simulink model "SIFT_final"  (R2015a)
settings: Solver=ode45  StartTime=0.0  StopTime=10.0  RelTol=1e-3
InitFcn:
  | %% DSPBuilder Start
  | alt_dspbuilder_update_model(bdroot)
  | %% DSPBuilder End
libraries: allblocks_alteradspbuilder2 x1826
(part 15 of 24)

== system SIFT_final/SIFT/SIFT_detector/Octave0/calculate_key_point/find_KeyPoint/find_Keymax ==
  dataIn_10 : Inport
  dataIn_11 : Inport  Port=2
  dataIn_12 : Inport  Port=3
  dataIn_13 : Inport  Port=4
  dataIn_14 : Inport  Port=5
  dataIn_15 : Inport  Port=6
  dataIn_16 : Inport  Port=7
  dataIn_17 : Inport  Port=8
  dataIn_18 : Inport  Port=9
  dataIn_20 : Inport  Port=10
  dataIn_21 : Inport  Port=11
  dataIn_22 : Inport  Port=12
  dataIn_23 : Inport  Port=13
  dataIn_24 : Inport  Port=14
  dataIn_25 : Inport  Port=15
  dataIn_26 : Inport  Port=16
  dataIn_27 : Inport  Port=17
  dataIn_28 : Inport  Port=18
  dataIn_30 : Inport  Port=19
  dataIn_31 : Inport  Port=20
  dataIn_32 : Inport  Port=21
  dataIn_33 : Inport  Port=22
  dataIn_34 : Inport  Port=23
  dataIn_35 : Inport  Port=24
  dataIn_36 : Inport  Port=25
  dataIn_37 : Inport  Port=26
  dataIn_38 : Inport  Port=27
  Comparator : allblocks_alteradspbuilder2/Comparator  direction=a > b  pipeline_display=0  allowFloatingPointOverride=on  logOutputs=off  logFile=G:\Project\SIFT 2octave\add frb\PCIE_Display\custom_ip\tb_SIFT\SIFT_SIFT_Subsystem_calculate%5Fkey%5Fpoint_find%5FKeyPoint_find%5FKeymax_Comparator.fixedpointlog
  Comparator1 : allblocks_alteradspbuilder2/Comparator  direction=a > b  pipeline_display=0  allowFloatingPointOverride=on  logOutputs=off  logFile=G:\Project\SIFT 2octave\add frb\PCIE_Display\custom_ip\tb_SIFT\SIFT_SIFT_Subsystem_calculate%5Fkey%5Fpoint_find%5FKeyPoint_find%5FKeymax_Comparator1.fixedpointlog
  Comparator10 : allblocks_alteradspbuilder2/Comparator  direction=a > b  pipeline_display=0  allowFloatingPointOverride=on  logOutputs=off  logFile=G:\Project\SIFT 2octave\add frb\PCIE_Display\custom_ip\tb_SIFT\SIFT_SIFT_Subsystem_calculate%5Fkey%5Fpoint_find%5FKeyPoint_find%5FKeymax_Comparator10.fixedpointlog
  Comparator11 : allblocks_alteradspbuilder2/Comparator  direction=a > b  pipeline_display=0  allowFloatingPointOverride=on  logOutputs=off  logFile=G:\Project\SIFT 2octave\add frb\PCIE_Display\custom_ip\tb_SIFT\SIFT_SIFT_Subsystem_calculate%5Fkey%5Fpoint_find%5FKeyPoint_find%5FKeymax_Comparator11.fixedpointlog
  Comparator12 : allblocks_alteradspbuilder2/Comparator  direction=a > b  pipeline_display=0  allowFloatingPointOverride=on  logOutputs=off  logFile=G:\Project\SIFT 2octave\add frb\PCIE_Display\custom_ip\tb_SIFT\SIFT_SIFT_Subsystem_calculate%5Fkey%5Fpoint_find%5FKeyPoint_find%5FKeymax_Comparator12.fixedpointlog
  Comparator13 : allblocks_alteradspbuilder2/Comparator  direction=a > b  pipeline_display=0  allowFloatingPointOverride=on  logOutputs=off  logFile=G:\Project\SIFT 2octave\add frb\PCIE_Display\custom_ip\tb_SIFT\SIFT_SIFT_Subsystem_calculate%5Fkey%5Fpoint_find%5FKeyPoint_find%5FKeymax_Comparator13.fixedpointlog
  Comparator14 : allblocks_alteradspbuilder2/Comparator  direction=a > b  pipeline_display=0  allowFloatingPointOverride=on  logOutputs=off  logFile=G:\Project\SIFT 2octave\add frb\PCIE_Display\custom_ip\tb_SIFT\SIFT_SIFT_Subsystem_calculate%5Fkey%5Fpoint_find%5FKeyPoint_find%5FKeymax_Comparator14.fixedpointlog
  Comparator15 : allblocks_alteradspbuilder2/Comparator  direction=a > b  pipeline_display=0  allowFloatingPointOverride=on  logOutputs=off  logFile=G:\Project\SIFT 2octave\add frb\PCIE_Display\custom_ip\tb_SIFT\SIFT_SIFT_Subsystem_calculate%5Fkey%5Fpoint_find%5FKeyPoint_find%5FKeymax_Comparator15.fixedpointlog
  Comparator16 : allblocks_alteradspbuilder2/Comparator  direction=a > b  pipeline_display=0  allowFloatingPointOverride=on  logOutputs=off  logFile=G:\Project\SIFT 2octave\add frb\PCIE_Display\custom_ip\tb_SIFT\SIFT_SIFT_Subsystem_calculate%5Fkey%5Fpoint_find%5FKeyPoint_find%5FKeymax_Comparator16.fixedpointlog
  Comparator17 : allblocks_alteradspbuilder2/Comparator  direction=a > b  pipeline_display=0  allowFloatingPointOverride=on  logOutputs=off  logFile=G:\Project\SIFT 2octave\add frb\PCIE_Display\custom_ip\tb_SIFT\SIFT_SIFT_Subsystem_calculate%5Fkey%5Fpoint_find%5FKeyPoint_find%5FKeymax_Comparator17.fixedpointlog
  Comparator19 : allblocks_alteradspbuilder2/Comparator  direction=a > b  pipeline_display=0  allowFloatingPointOverride=on  logOutputs=off  logFile=G:\Project\SIFT 2octave\add frb\PCIE_Display\custom_ip\tb_SIFT\SIFT_SIFT_Subsystem_calculate%5Fkey%5Fpoint_find%5FKeyPoint_find%5FKeymax_Comparator19.fixedpointlog
  Comparator2 : allblocks_alteradspbuilder2/Comparator  direction=a > b  pipeline_display=0  allowFloatingPointOverride=on  logOutputs=off  logFile=G:\Project\SIFT 2octave\add frb\PCIE_Display\custom_ip\tb_SIFT\SIFT_SIFT_Subsystem_calculate%5Fkey%5Fpoint_find%5FKeyPoint_find%5FKeymax_Comparator2.fixedpointlog
  Comparator20 : allblocks_alteradspbuilder2/Comparator  direction=a > b  pipeline_display=0  allowFloatingPointOverride=on  logOutputs=off  logFile=G:\Project\SIFT 2octave\add frb\PCIE_Display\custom_ip\tb_SIFT\SIFT_SIFT_Subsystem_calculate%5Fkey%5Fpoint_find%5FKeyPoint_find%5FKeymax_Comparator20.fixedpointlog
  Comparator27 : allblocks_alteradspbuilder2/Comparator  direction=a > b  pipeline_display=0  allowFloatingPointOverride=on  logOutputs=off  logFile=G:\Project\SIFT 2octave\add frb\PCIE_Display\custom_ip\tb_SIFT\SIFT_SIFT_Subsystem_calculate%5Fkey%5Fpoint_find%5FKeyPoint_find%5FKeymax_Comparator27.fixedpointlog
  Comparator28 : allblocks_alteradspbuilder2/Comparator  direction=a > b  pipeline_display=0  allowFloatingPointOverride=on  logOutputs=off  logFile=G:\Project\SIFT 2octave\add frb\PCIE_Display\custom_ip\tb_SIFT\SIFT_SIFT_Subsystem_calculate%5Fkey%5Fpoint_find%5FKeyPoint_find%5FKeymax_Comparator28.fixedpointlog
  Comparator29 : allblocks_alteradspbuilder2/Comparator  direction=a > b  pipeline_display=0  allowFloatingPointOverride=on  logOutputs=off  logFile=G:\Project\SIFT 2octave\add frb\PCIE_Display\custom_ip\tb_SIFT\SIFT_SIFT_Subsystem_calculate%5Fkey%5Fpoint_find%5FKeyPoint_find%5FKeymax_Comparator29.fixedpointlog
  Comparator3 : allblocks_alteradspbuilder2/Comparator  direction=a > b  pipeline_display=0  allowFloatingPointOverride=on  logOutputs=off  logFile=G:\Project\SIFT 2octave\add frb\PCIE_Display\custom_ip\tb_SIFT\SIFT_SIFT_Subsystem_calculate%5Fkey%5Fpoint_find%5FKeyPoint_find%5FKeymax_Comparator3.fixedpointlog
  Comparator30 : allblocks_alteradspbuilder2/Comparator  direction=a > b  pipeline_display=0  allowFloatingPointOverride=on  logOutputs=off  logFile=G:\Project\SIFT 2octave\add frb\PCIE_Display\custom_ip\tb_SIFT\SIFT_SIFT_Subsystem_calculate%5Fkey%5Fpoint_find%5FKeyPoint_find%5FKeymax_Comparator30.fixedpointlog
  Comparator31 : allblocks_alteradspbuilder2/Comparator  direction=a > b  pipeline_display=0  allowFloatingPointOverride=on  logOutputs=off  logFile=G:\Project\SIFT 2octave\add frb\PCIE_Display\custom_ip\tb_SIFT\SIFT_SIFT_Subsystem_calculate%5Fkey%5Fpoint_find%5FKeyPoint_find%5FKeymax_Comparator31.fixedpointlog
  Comparator32 : allblocks_alteradspbuilder2/Comparator  direction=a > b  pipeline_display=0  allowFloatingPointOverride=on  logOutputs=off  logFile=G:\Project\SIFT 2octave\add frb\PCIE_Display\custom_ip\tb_SIFT\SIFT_SIFT_Subsystem_calculate%5Fkey%5Fpoint_find%5FKeyPoint_find%5FKeymax_Comparator32.fixedpointlog
  Comparator33 : allblocks_alteradspbuilder2/Comparator  direction=a > b  pipeline_display=0  allowFloatingPointOverride=on  logOutputs=off  logFile=G:\Project\SIFT 2octave\add frb\PCIE_Display\custom_ip\tb_SIFT\SIFT_SIFT_Subsystem_calculate%5Fkey%5Fpoint_find%5FKeyPoint_find%5FKeymax_Comparator33.fixedpointlog
  Comparator34 : allblocks_alteradspbuilder2/Comparator  direction=a > b  pipeline_display=0  allowFloatingPointOverride=on  logOutputs=off  logFile=G:\Project\SIFT 2octave\add frb\PCIE_Display\custom_ip\tb_SIFT\SIFT_SIFT_Subsystem_calculate%5Fkey%5Fpoint_find%5FKeyPoint_find%5FKeymax_Comparator34.fixedpointlog
  Comparator35 : allblocks_alteradspbuilder2/Comparator  direction=a > b  pipeline_display=0  allowFloatingPointOverride=on  logOutputs=off  logFile=G:\Project\SIFT 2octave\add frb\PCIE_Display\custom_ip\tb_SIFT\SIFT_SIFT_Subsystem_calculate%5Fkey%5Fpoint_find%5FKeyPoint_find%5FKeymax_Comparator35.fixedpointlog
  Comparator4 : allblocks_alteradspbuilder2/Comparator  direction=a > b  pipeline_display=0  allowFloatingPointOverride=on  logOutputs=off  logFile=G:\Project\SIFT 2octave\add frb\PCIE_Display\custom_ip\tb_SIFT\SIFT_SIFT_Subsystem_calculate%5Fkey%5Fpoint_find%5FKeyPoint_find%5FKeymax_Comparator4.fixedpointlog
  Comparator5 : allblocks_alteradspbuilder2/Comparator  direction=a > b  pipeline_display=0  allowFloatingPointOverride=on  logOutputs=off  logFile=G:\Project\SIFT 2octave\add frb\PCIE_Display\custom_ip\tb_SIFT\SIFT_SIFT_Subsystem_calculate%5Fkey%5Fpoint_find%5FKeyPoint_find%5FKeymax_Comparator5.fixedpointlog
  Comparator6 : allblocks_alteradspbuilder2/Comparator  direction=a < b  pipeline_display=0  allowFloatingPointOverride=on  logOutputs=off  logFile=G:\Project\SIFT 2octave\add frb\PCIE_Display\custom_ip\tb_SIFT\SIFT_SIFT_Subsystem_calculate%5Fkey%5Fpoint_find%5FKeyPoint_find%5FKeymax_Comparator6.fixedpointlog
  Comparator7 : allblocks_alteradspbuilder2/Comparator  direction=a < b  pipeline_display=0  allowFloatingPointOverride=on  logOutputs=off  logFile=G:\Project\SIFT 2octave\add frb\PCIE_Display\custom_ip\tb_SIFT\SIFT_SIFT_Subsystem_calculate%5Fkey%5Fpoint_find%5FKeyPoint_find%5FKeymax_Comparator7.fixedpointlog
  Comparator9 : allblocks_alteradspbuilder2/Comparator  direction=a > b  pipeline_display=0  allowFloatingPointOverride=on  logOutputs=off  logFile=G:\Project\SIFT 2octave\add frb\PCIE_Display\custom_ip\tb_SIFT\SIFT_SIFT_Subsystem_calculate%5Fkey%5Fpoint_find%5FKeyPoint_find%5FKeymax_Comparator9.fixedpointlog
  Constant : allblocks_alteradspbuilder2/Constant  mask_cst=0.8*0.015  BusType=Signed Fractional  bwl=9  bwr=16  roundMode=Truncate  satMode=Wrap  SpecifyClock=off  allowFloatingPointOverride=on  logOutputs=off  logFile=G:\Project\SIFT 2octave\add frb\PCIE_Display\custom_ip\tb_SIFT\SIFT_SIFT_Subsystem_calculate%5Fkey%5Fpoint_find%5FKeyPoint_find%5FKeymax_Constant.fixedpointlog
  Constant1 : allblocks_alteradspbuilder2/Constant  mask_cst=-0.8*0.015  BusType=Signed Fractional  bwl=9  bwr=16  roundMode=Truncate  satMode=Wrap  SpecifyClock=off  allowFloatingPointOverride=on  logOutputs=off  logFile=G:\Project\SIFT 2octave\add frb\PCIE_Display\custom_ip\tb_SIFT\SIFT_SIFT_Subsystem_calculate%5Fkey%5Fpoint_find%5FKeyPoint_find%5FKeymax_Constant1.fixedpointlog
  Logical Bit Operator : allblocks_alteradspbuilder2/Logical Bit Operator  LogicalOperator=OR  user_inputs=2  pipeline_display=0
  Logical Bit Operator2 : allblocks_alteradspbuilder2/Logical Bit Operator  LogicalOperator=AND  user_inputs=27  pipeline_display=0
  is_KeyPoint : Outport
  wires:
  dataIn_18/1 -> [dataIn_18]
  dataIn_10/1 -> [dataIn_10]
  [result_10] -> Logical Bit Operator2/1
  [dataIn_24] -> Comparator/1
  Comparator1/1 -> [result_11]
  [dataIn_10] -> Comparator/2
  [dataIn_24] -> Comparator1/1
  [dataIn_11] -> Comparator1/2
  [result_20] -> Logical Bit Operator2/10
  [result_11] -> Logical Bit Operator2/2
  [result_22] -> Logical Bit Operator2/12
  [result_23] -> Logical Bit Operator2/13
  Comparator7/1 -> Logical Bit Operator/2
  [dataIn_24] -> Comparator2/1
  [dataIn_24] -> Comparator6/2
  Comparator2/1 -> [result_12]
  [dataIn_12] -> Comparator2/2
  [result_21] -> Logical Bit Operator2/11
  [dataIn_24] -> Comparator9/1
  Comparator9/1 -> [result_16]
  [dataIn_24] -> Comparator10/1
  [dataIn_16] -> Comparator9/2
  Comparator10/1 -> [result_17]
  [dataIn_17] -> Comparator10/2
  [dataIn_24] -> Comparator11/1
  Comparator11/1 -> [result_18]
  [dataIn_18] -> Comparator11/2
  dataIn_14/1 -> [dataIn_14]
  dataIn_15/1 -> [dataIn_15]
  dataIn_17/1 -> [dataIn_17]
  dataIn_16/1 -> [dataIn_16]
  dataIn_24/1 -> [dataIn_24]
  dataIn_27/1 -> [dataIn_27]
  dataIn_28/1 -> [dataIn_28]
  dataIn_25/1 -> [dataIn_25]
  dataIn_22/1 -> [dataIn_22]
  dataIn_20/1 -> [dataIn_20]
  dataIn_21/1 -> [dataIn_21]
  dataIn_23/1 -> [dataIn_23]
  dataIn_26/1 -> [dataIn_26]
  dataIn_30/1 -> [dataIn_30]
  dataIn_31/1 -> [dataIn_31]
  dataIn_32/1 -> [dataIn_32]
  dataIn_33/1 -> [dataIn_33]
  dataIn_37/1 -> [dataIn_37]
  dataIn_35/1 -> [dataIn_35]
  dataIn_34/1 -> [dataIn_34]
  dataIn_36/1 -> [dataIn_36]
  dataIn_38/1 -> [dataIn_38]
  dataIn_11/1 -> [dataIn_11]
  [dataIn_24] -> Comparator7/1
  [dataIn_13] -> Comparator3/2
  Comparator3/1 -> [result_13]
  [dataIn_24] -> Comparator4/1
  [dataIn_24] -> Comparator3/1
  [dataIn_24] -> Comparator5/1
  Comparator5/1 -> [result_15]
  [dataIn_14] -> Comparator4/2
  [dataIn_15] -> Comparator5/2
  Comparator4/1 -> [result_14]
  [dataIn_24] -> Comparator27/1
  [dataIn_24] -> Comparator28/1
  [dataIn_24] -> Comparator31/1
  [dataIn_32] -> Comparator31/2
  [dataIn_24] -> Comparator32/1
  [dataIn_33] -> Comparator32/2
  [dataIn_24] -> Comparator33/1
  Comparator32/1 -> [result_33]
  Comparator27/1 -> [result_30]
  Comparator28/1 -> [result_31]
  Comparator31/1 -> [result_32]
  [dataIn_30] -> Comparator27/2
  [dataIn_31] -> Comparator28/2
  [dataIn_35] -> Comparator34/2
  Comparator35/1 -> [result_36]
  Comparator34/1 -> [result_35]
  [dataIn_34] -> Comparator33/2
  [dataIn_24] -> Comparator35/1
  Comparator29/1 -> [result_37]
  [dataIn_24] -> Comparator30/1
  [dataIn_36] -> Comparator35/2
  Comparator30/1 -> [result_38]
  [dataIn_24] -> Comparator34/1
  [dataIn_24] -> Comparator29/1
  [dataIn_37] -> Comparator29/2
  [dataIn_38] -> Comparator30/2
  Comparator33/1 -> [result_34]
  [result_13] -> Logical Bit Operator2/4
  [result_17] -> Logical Bit Operator2/8
  [result_14] -> Logical Bit Operator2/5
  [result_15] -> Logical Bit Operator2/6
  [result_16] -> Logical Bit Operator2/7
  [result_18] -> Logical Bit Operator2/9
  [result_12] -> Logical Bit Operator2/3
  Constant/1 -> Comparator6/1
  Logical Bit Operator/1 -> [result_24]
  Logical Bit Operator2/1 -> [isKeyPoint]
  Constant1/1 -> Comparator7/2
  Comparator6/1 -> Logical Bit Operator/1
  [dataIn_24] -> Comparator12/1
  [dataIn_25] -> Comparator19/2
  Comparator13/1 -> [result_21]
  Comparator19/1 -> [result_25]
  [dataIn_24] -> Comparator19/1
  [dataIn_20] -> Comparator12/2
  [dataIn_24] -> Comparator16/1
  [dataIn_24] -> Comparator14/1
  [dataIn_24] -> Comparator13/1
  Comparator16/1 -> [result_22]
  [dataIn_22] -> Comparator16/2
  Comparator14/1 -> [result_27]
  [dataIn_24] -> Comparator17/1
  [dataIn_23] -> Comparator17/2
  [dataIn_24] -> Comparator15/1
  [dataIn_27] -> Comparator14/2
  Comparator17/1 -> [result_23]
  [dataIn_28] -> Comparator15/2
  [dataIn_26] -> Comparator20/2
  Comparator12/1 -> [result_20]
  [dataIn_24] -> Comparator20/1
  Comparator15/1 -> [result_28]
  Comparator20/1 -> [result_26]
  [dataIn_21] -> Comparator13/2
  [isKeyPoint] -> is_KeyPoint/1
  dataIn_12/1 -> [dataIn_12]
  dataIn_13/1 -> [dataIn_13]
  Comparator/1 -> [result_10]
  [result_28] -> Logical Bit Operator2/18
  [result_30] -> Logical Bit Operator2/19
  [result_31] -> Logical Bit Operator2/20
  [result_33] -> Logical Bit Operator2/22
  [result_34] -> Logical Bit Operator2/23
  [result_36] -> Logical Bit Operator2/25
  [result_35] -> Logical Bit Operator2/24
  [result_32] -> Logical Bit Operator2/21
  [result_37] -> Logical Bit Operator2/26
  [result_38] -> Logical Bit Operator2/27
  [result_26] -> Logical Bit Operator2/16
  [result_25] -> Logical Bit Operator2/15
  [result_27] -> Logical Bit Operator2/17
  [result_24] -> Logical Bit Operator2/14

== system SIFT_final/SIFT/SIFT_detector/Octave0/calculate_key_point/find_KeyPoint/find_min ==
  dataIn_10 : Inport
  dataIn_11 : Inport  Port=2
  dataIn_12 : Inport  Port=3
  dataIn_13 : Inport  Port=4
  dataIn_14 : Inport  Port=5
  dataIn_15 : Inport  Port=6
  dataIn_16 : Inport  Port=7
  dataIn_17 : Inport  Port=8
  dataIn_18 : Inport  Port=9
  dataIn_20 : Inport  Port=10
  dataIn_21 : Inport  Port=11
  dataIn_22 : Inport  Port=12
  dataIn_23 : Inport  Port=13
  dataIn_24 : Inport  Port=14
  dataIn_25 : Inport  Port=15
  dataIn_26 : Inport  Port=16
  dataIn_27 : Inport  Port=17
  dataIn_28 : Inport  Port=18
  dataIn_30 : Inport  Port=19
  dataIn_31 : Inport  Port=20
  dataIn_32 : Inport  Port=21
  dataIn_33 : Inport  Port=22
  dataIn_34 : Inport  Port=23
  dataIn_35 : Inport  Port=24
  dataIn_36 : Inport  Port=25
  dataIn_37 : Inport  Port=26
  dataIn_38 : Inport  Port=27
  Comparator : allblocks_alteradspbuilder2/Comparator  direction=a < b  pipeline_display=0  allowFloatingPointOverride=on  logOutputs=off  logFile=G:\Project\SIFT 2octave\add frb\PCIE_Display\custom_ip\tb_SIFT\SIFT_SIFT_Subsystem_calculate%5Fkey%5Fpoint_find%5FKeyPoint_find%5Fmin_Comparator.fixedpointlog
  Comparator1 : allblocks_alteradspbuilder2/Comparator  direction=a < b  pipeline_display=0  allowFloatingPointOverride=on  logOutputs=off  logFile=G:\Project\SIFT 2octave\add frb\PCIE_Display\custom_ip\tb_SIFT\SIFT_SIFT_Subsystem_calculate%5Fkey%5Fpoint_find%5FKeyPoint_find%5Fmin_Comparator1.fixedpointlog
  Comparator10 : allblocks_alteradspbuilder2/Comparator  direction=a < b  pipeline_display=0  allowFloatingPointOverride=on  logOutputs=off  logFile=G:\Project\SIFT 2octave\add frb\PCIE_Display\custom_ip\tb_SIFT\SIFT_SIFT_Subsystem_calculate%5Fkey%5Fpoint_find%5FKeyPoint_find%5Fmin_Comparator10.fixedpointlog
  Comparator11 : allblocks_alteradspbuilder2/Comparator  direction=a < b  pipeline_display=0  allowFloatingPointOverride=on  logOutputs=off  logFile=G:\Project\SIFT 2octave\add frb\PCIE_Display\custom_ip\tb_SIFT\SIFT_SIFT_Subsystem_calculate%5Fkey%5Fpoint_find%5FKeyPoint_find%5Fmin_Comparator11.fixedpointlog
  Comparator12 : allblocks_alteradspbuilder2/Comparator  direction=a < b  pipeline_display=0  allowFloatingPointOverride=on  logOutputs=off  logFile=G:\Project\SIFT 2octave\add frb\PCIE_Display\custom_ip\tb_SIFT\SIFT_SIFT_Subsystem_calculate%5Fkey%5Fpoint_find%5FKeyPoint_find%5Fmin_Comparator12.fixedpointlog
  Comparator13 : allblocks_alteradspbuilder2/Comparator  direction=a < b  pipeline_display=0  allowFloatingPointOverride=on  logOutputs=off  logFile=G:\Project\SIFT 2octave\add frb\PCIE_Display\custom_ip\tb_SIFT\SIFT_SIFT_Subsystem_calculate%5Fkey%5Fpoint_find%5FKeyPoint_find%5Fmin_Comparator13.fixedpointlog
  Comparator14 : allblocks_alteradspbuilder2/Comparator  direction=a < b  pipeline_display=0  allowFloatingPointOverride=on  logOutputs=off  logFile=G:\Project\SIFT 2octave\add frb\PCIE_Display\custom_ip\tb_SIFT\SIFT_SIFT_Subsystem_calculate%5Fkey%5Fpoint_find%5FKeyPoint_find%5Fmin_Comparator14.fixedpointlog
  Comparator15 : allblocks_alteradspbuilder2/Comparator  direction=a < b  pipeline_display=0  allowFloatingPointOverride=on  logOutputs=off  logFile=G:\Project\SIFT 2octave\add frb\PCIE_Display\custom_ip\tb_SIFT\SIFT_SIFT_Subsystem_calculate%5Fkey%5Fpoint_find%5FKeyPoint_find%5Fmin_Comparator15.fixedpointlog
  Comparator16 : allblocks_alteradspbuilder2/Comparator  direction=a < b  pipeline_display=0  allowFloatingPointOverride=on  logOutputs=off  logFile=G:\Project\SIFT 2octave\add frb\PCIE_Display\custom_ip\tb_SIFT\SIFT_SIFT_Subsystem_calculate%5Fkey%5Fpoint_find%5FKeyPoint_find%5Fmin_Comparator16.fixedpointlog
  Comparator17 : allblocks_alteradspbuilder2/Comparator  direction=a < b  pipeline_display=0  allowFloatingPointOverride=on  logOutputs=off  logFile=G:\Project\SIFT 2octave\add frb\PCIE_Display\custom_ip\tb_SIFT\SIFT_SIFT_Subsystem_calculate%5Fkey%5Fpoint_find%5FKeyPoint_find%5Fmin_Comparator17.fixedpointlog
  Comparator19 : allblocks_alteradspbuilder2/Comparator  direction=a < b  pipeline_display=0  allowFloatingPointOverride=on  logOutputs=off  logFile=G:\Project\SIFT 2octave\add frb\PCIE_Display\custom_ip\tb_SIFT\SIFT_SIFT_Subsystem_calculate%5Fkey%5Fpoint_find%5FKeyPoint_find%5Fmin_Comparator19.fixedpointlog
  Comparator2 : allblocks_alteradspbuilder2/Comparator  direction=a < b  pipeline_display=0  allowFloatingPointOverride=on  logOutputs=off  logFile=G:\Project\SIFT 2octave\add frb\PCIE_Display\custom_ip\tb_SIFT\SIFT_SIFT_Subsystem_calculate%5Fkey%5Fpoint_find%5FKeyPoint_find%5Fmin_Comparator2.fixedpointlog
  Comparator20 : allblocks_alteradspbuilder2/Comparator  direction=a < b  pipeline_display=0  allowFloatingPointOverride=on  logOutputs=off  logFile=G:\Project\SIFT 2octave\add frb\PCIE_Display\custom_ip\tb_SIFT\SIFT_SIFT_Subsystem_calculate%5Fkey%5Fpoint_find%5FKeyPoint_find%5Fmin_Comparator20.fixedpointlog
  Comparator27 : allblocks_alteradspbuilder2/Comparator  direction=a < b  pipeline_display=0  allowFloatingPointOverride=on  logOutputs=off  logFile=G:\Project\SIFT 2octave\add frb\PCIE_Display\custom_ip\tb_SIFT\SIFT_SIFT_Subsystem_calculate%5Fkey%5Fpoint_find%5FKeyPoint_find%5Fmin_Comparator27.fixedpointlog
  Comparator28 : allblocks_alteradspbuilder2/Comparator  direction=a < b  pipeline_display=0  allowFloatingPointOverride=on  logOutputs=off  logFile=G:\Project\SIFT 2octave\add frb\PCIE_Display\custom_ip\tb_SIFT\SIFT_SIFT_Subsystem_calculate%5Fkey%5Fpoint_find%5FKeyPoint_find%5Fmin_Comparator28.fixedpointlog
  Comparator29 : allblocks_alteradspbuilder2/Comparator  direction=a < b  pipeline_display=0  allowFloatingPointOverride=on  logOutputs=off  logFile=G:\Project\SIFT 2octave\add frb\PCIE_Display\custom_ip\tb_SIFT\SIFT_SIFT_Subsystem_calculate%5Fkey%5Fpoint_find%5FKeyPoint_find%5Fmin_Comparator29.fixedpointlog
  Comparator3 : allblocks_alteradspbuilder2/Comparator  direction=a < b  pipeline_display=0  allowFloatingPointOverride=on  logOutputs=off  logFile=G:\Project\SIFT 2octave\add frb\PCIE_Display\custom_ip\tb_SIFT\SIFT_SIFT_Subsystem_calculate%5Fkey%5Fpoint_find%5FKeyPoint_find%5Fmin_Comparator3.fixedpointlog
  Comparator30 : allblocks_alteradspbuilder2/Comparator  direction=a < b  pipeline_display=0  allowFloatingPointOverride=on  logOutputs=off  logFile=G:\Project\SIFT 2octave\add frb\PCIE_Display\custom_ip\tb_SIFT\SIFT_SIFT_Subsystem_calculate%5Fkey%5Fpoint_find%5FKeyPoint_find%5Fmin_Comparator30.fixedpointlog
  Comparator31 : allblocks_alteradspbuilder2/Comparator  direction=a < b  pipeline_display=0  allowFloatingPointOverride=on  logOutputs=off  logFile=G:\Project\SIFT 2octave\add frb\PCIE_Display\custom_ip\tb_SIFT\SIFT_SIFT_Subsystem_calculate%5Fkey%5Fpoint_find%5FKeyPoint_find%5Fmin_Comparator31.fixedpointlog
  Comparator32 : allblocks_alteradspbuilder2/Comparator  direction=a < b  pipeline_display=0  allowFloatingPointOverride=on  logOutputs=off  logFile=G:\Project\SIFT 2octave\add frb\PCIE_Display\custom_ip\tb_SIFT\SIFT_SIFT_Subsystem_calculate%5Fkey%5Fpoint_find%5FKeyPoint_find%5Fmin_Comparator32.fixedpointlog
  Comparator33 : allblocks_alteradspbuilder2/Comparator  direction=a < b  pipeline_display=0  allowFloatingPointOverride=on  logOutputs=off  logFile=G:\Project\SIFT 2octave\add frb\PCIE_Display\custom_ip\tb_SIFT\SIFT_SIFT_Subsystem_calculate%5Fkey%5Fpoint_find%5FKeyPoint_find%5Fmin_Comparator33.fixedpointlog
  Comparator34 : allblocks_alteradspbuilder2/Comparator  direction=a < b  pipeline_display=0  allowFloatingPointOverride=on  logOutputs=off  logFile=G:\Project\SIFT 2octave\add frb\PCIE_Display\custom_ip\tb_SIFT\SIFT_SIFT_Subsystem_calculate%5Fkey%5Fpoint_find%5FKeyPoint_find%5Fmin_Comparator34.fixedpointlog
  Comparator35 : allblocks_alteradspbuilder2/Comparator  direction=a < b  pipeline_display=0  allowFloatingPointOverride=on  logOutputs=off  logFile=G:\Project\SIFT 2octave\add frb\PCIE_Display\custom_ip\tb_SIFT\SIFT_SIFT_Subsystem_calculate%5Fkey%5Fpoint_find%5FKeyPoint_find%5Fmin_Comparator35.fixedpointlog
  Comparator4 : allblocks_alteradspbuilder2/Comparator  direction=a < b  pipeline_display=0  allowFloatingPointOverride=on  logOutputs=off  logFile=G:\Project\SIFT 2octave\add frb\PCIE_Display\custom_ip\tb_SIFT\SIFT_SIFT_Subsystem_calculate%5Fkey%5Fpoint_find%5FKeyPoint_find%5Fmin_Comparator4.fixedpointlog
  Comparator5 : allblocks_alteradspbuilder2/Comparator  direction=a < b  pipeline_display=0  allowFloatingPointOverride=on  logOutputs=off  logFile=G:\Project\SIFT 2octave\add frb\PCIE_Display\custom_ip\tb_SIFT\SIFT_SIFT_Subsystem_calculate%5Fkey%5Fpoint_find%5FKeyPoint_find%5Fmin_Comparator5.fixedpointlog
  Comparator6 : allblocks_alteradspbuilder2/Comparator  direction=a < b  pipeline_display=0  allowFloatingPointOverride=on  logOutputs=off  logFile=G:\Project\SIFT 2octave\add frb\PCIE_Display\custom_ip\tb_SIFT\SIFT_SIFT_Subsystem_calculate%5Fkey%5Fpoint_find%5FKeyPoint_find%5Fmin_Comparator6.fixedpointlog
  Comparator7 : allblocks_alteradspbuilder2/Comparator  direction=a < b  pipeline_display=0  allowFloatingPointOverride=on  logOutputs=off  logFile=G:\Project\SIFT 2octave\add frb\PCIE_Display\custom_ip\tb_SIFT\SIFT_SIFT_Subsystem_calculate%5Fkey%5Fpoint_find%5FKeyPoint_find%5Fmin_Comparator7.fixedpointlog
  Comparator9 : allblocks_alteradspbuilder2/Comparator  direction=a < b  pipeline_display=0  allowFloatingPointOverride=on  logOutputs=off  logFile=G:\Project\SIFT 2octave\add frb\PCIE_Display\custom_ip\tb_SIFT\SIFT_SIFT_Subsystem_calculate%5Fkey%5Fpoint_find%5FKeyPoint_find%5Fmin_Comparator9.fixedpointlog
  Constant : allblocks_alteradspbuilder2/Constant  mask_cst=0.8*0.015  BusType=Signed Fractional  bwl=9  bwr=16  roundMode=Truncate  satMode=Wrap  SpecifyClock=off  allowFloatingPointOverride=on  logOutputs=off  logFile=G:\Project\SIFT 2octave\add frb\PCIE_Display\custom_ip\tb_SIFT\SIFT_SIFT_Subsystem_calculate%5Fkey%5Fpoint_find%5FKeyPoint_find%5Fmin_Constant.fixedpointlog
  Constant1 : allblocks_alteradspbuilder2/Constant  mask_cst=-0.8*0.015  BusType=Signed Fractional  bwl=9  bwr=16  roundMode=Truncate  satMode=Wrap  SpecifyClock=off  allowFloatingPointOverride=on  logOutputs=off  logFile=G:\Project\SIFT 2octave\add frb\PCIE_Display\custom_ip\tb_SIFT\SIFT_SIFT_Subsystem_calculate%5Fkey%5Fpoint_find%5FKeyPoint_find%5Fmin_Constant1.fixedpointlog
  Logical Bit Operator : allblocks_alteradspbuilder2/Logical Bit Operator  LogicalOperator=OR  user_inputs=2  pipeline_display=0
  Logical Bit Operator2 : allblocks_alteradspbuilder2/Logical Bit Operator  LogicalOperator=AND  user_inputs=27  pipeline_display=0
  is_KeyPoint : Outport
  wires:
  dataIn_18/1 -> [dataIn_18]
  dataIn_10/1 -> [dataIn_10]
  [result_10] -> Logical Bit Operator2/1
  [dataIn_24] -> Comparator/1
  Comparator1/1 -> [result_11]
  [dataIn_10] -> Comparator/2
  [dataIn_24] -> Comparator1/1
  [dataIn_11] -> Comparator1/2
  [result_20] -> Logical Bit Operator2/10
  [result_11] -> Logical Bit Operator2/2
  [result_22] -> Logical Bit Operator2/12
  [result_23] -> Logical Bit Operator2/13
  Comparator7/1 -> Logical Bit Operator/2
  [dataIn_24] -> Comparator2/1
  [dataIn_24] -> Comparator6/2
  Comparator2/1 -> [result_12]
  [dataIn_12] -> Comparator2/2
  [result_21] -> Logical Bit Operator2/11
  [dataIn_24] -> Comparator9/1
  Comparator9/1 -> [result_16]
  [dataIn_24] -> Comparator10/1
  [dataIn_16] -> Comparator9/2
  Comparator10/1 -> [result_17]
  [dataIn_17] -> Comparator10/2
  [dataIn_24] -> Comparator11/1
  Comparator11/1 -> [result_18]
  [dataIn_18] -> Comparator11/2
  dataIn_14/1 -> [dataIn_14]
  dataIn_15/1 -> [dataIn_15]
  dataIn_17/1 -> [dataIn_17]
  dataIn_16/1 -> [dataIn_16]
  dataIn_24/1 -> [dataIn_24]
  dataIn_27/1 -> [dataIn_27]
  dataIn_28/1 -> [dataIn_28]
  dataIn_25/1 -> [dataIn_25]
  dataIn_22/1 -> [dataIn_22]
  dataIn_20/1 -> [dataIn_20]
  dataIn_21/1 -> [dataIn_21]
  dataIn_23/1 -> [dataIn_23]
  dataIn_26/1 -> [dataIn_26]
  dataIn_30/1 -> [dataIn_30]
  dataIn_31/1 -> [dataIn_31]
  dataIn_32/1 -> [dataIn_32]
  dataIn_33/1 -> [dataIn_33]
  dataIn_37/1 -> [dataIn_37]
  dataIn_35/1 -> [dataIn_35]
  dataIn_34/1 -> [dataIn_34]
  dataIn_36/1 -> [dataIn_36]
  dataIn_38/1 -> [dataIn_38]
  dataIn_11/1 -> [dataIn_11]
  [dataIn_24] -> Comparator7/1
  [dataIn_13] -> Comparator3/2
  Comparator3/1 -> [result_13]
  [dataIn_24] -> Comparator4/1
  [dataIn_24] -> Comparator3/1
  [dataIn_24] -> Comparator5/1
  Comparator5/1 -> [result_15]
  [dataIn_14] -> Comparator4/2
  [dataIn_15] -> Comparator5/2
  Comparator4/1 -> [result_14]
  [dataIn_24] -> Comparator27/1
  [dataIn_24] -> Comparator28/1
  [dataIn_24] -> Comparator31/1
  [dataIn_32] -> Comparator31/2
  [dataIn_24] -> Comparator32/1
  [dataIn_33] -> Comparator32/2
  [dataIn_24] -> Comparator33/1
  Comparator32/1 -> [result_33]
  Comparator27/1 -> [result_30]
  Comparator28/1 -> [result_31]
  Comparator31/1 -> [result_32]
  [dataIn_30] -> Comparator27/2
  [dataIn_31] -> Comparator28/2
  [dataIn_35] -> Comparator34/2
  Comparator35/1 -> [result_36]
  Comparator34/1 -> [result_35]
  [dataIn_34] -> Comparator33/2
  [dataIn_24] -> Comparator35/1
  Comparator29/1 -> [result_37]
  [dataIn_24] -> Comparator30/1
  [dataIn_36] -> Comparator35/2
  Comparator30/1 -> [result_38]
  [dataIn_24] -> Comparator34/1
  [dataIn_24] -> Comparator29/1
  [dataIn_37] -> Comparator29/2
  [dataIn_38] -> Comparator30/2
  Comparator33/1 -> [result_34]
  [result_13] -> Logical Bit Operator2/4
  [result_17] -> Logical Bit Operator2/8
  [result_14] -> Logical Bit Operator2/5
  [result_15] -> Logical Bit Operator2/6
  [result_16] -> Logical Bit Operator2/7
  [result_18] -> Logical Bit Operator2/9
  [result_12] -> Logical Bit Operator2/3
  Constant/1 -> Comparator6/1
  Logical Bit Operator/1 -> [result_24]
  Constant1/1 -> Comparator7/2
  Comparator6/1 -> Logical Bit Operator/1
  [dataIn_24] -> Comparator12/1
  [dataIn_25] -> Comparator19/2
  Comparator13/1 -> [result_21]
  Comparator19/1 -> [result_25]
  [dataIn_24] -> Comparator19/1
  [dataIn_20] -> Comparator12/2
  [dataIn_24] -> Comparator16/1
  [dataIn_24] -> Comparator14/1
  [dataIn_24] -> Comparator13/1
  Comparator16/1 -> [result_22]
  [dataIn_22] -> Comparator16/2
  Comparator14/1 -> [result_27]
  [dataIn_24] -> Comparator17/1
  [dataIn_23] -> Comparator17/2
  [dataIn_24] -> Comparator15/1
  [dataIn_27] -> Comparator14/2
  Comparator17/1 -> [result_23]
  [dataIn_28] -> Comparator15/2
  [dataIn_26] -> Comparator20/2
  Comparator12/1 -> [result_20]
  [dataIn_24] -> Comparator20/1
  Comparator15/1 -> [result_28]
  Comparator20/1 -> [result_26]
  [dataIn_21] -> Comparator13/2
  [isKeyPoint] -> is_KeyPoint/1
  dataIn_12/1 -> [dataIn_12]
  dataIn_13/1 -> [dataIn_13]
  Comparator/1 -> [result_10]
  [result_28] -> Logical Bit Operator2/18
  [result_30] -> Logical Bit Operator2/19
  [result_31] -> Logical Bit Operator2/20
  [result_33] -> Logical Bit Operator2/22
  [result_34] -> Logical Bit Operator2/23
  [result_36] -> Logical Bit Operator2/25
  [result_35] -> Logical Bit Operator2/24
  [result_32] -> Logical Bit Operator2/21
  [result_37] -> Logical Bit Operator2/26
  [result_38] -> Logical Bit Operator2/27
  [result_26] -> Logical Bit Operator2/16
  [result_25] -> Logical Bit Operator2/15
  [result_27] -> Logical Bit Operator2/17
  [result_24] -> Logical Bit Operator2/14
  Logical Bit Operator2/1 -> [isKeyPoint]
